simulink library "Vapour_Pressure"  (Simulink 8.2)
settings: Solver=ode45  StartTime=0.0  StopTime=10.0  RelTol=1e-3
undefined symbols (not defined in the file): CarnotCallbacks_Vapour_Pressure
settings Model: Creator=lena.frank  LastModifiedBy=drhf

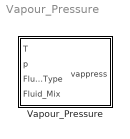
== system Vapour_Pressure ==
  Vapour_Pressure : Subsystem  LoadFcn=CarnotCallbacks_Vapour_Pressure('LoadFcn');  InitFcn=load('THB.mat');  VariantControl=CarlibClassic  mask(vapourpressure){INPUTARGUMENTS=state variables (classic), DEBUGLEVEL=WARNINGLEVEL, MAXTOTALMESSAGES=inf, MAXCONSECUTIVEMESSAGES=inf, WRITETOFILE=0, FILENAME='errors.txt'}
      mask prompts: INPUTARGUMENTS "Input arguments"; DEBUGLEVEL "Debug level"; MAXTOTALMESSAGES "maximum number of total warning"; MAXCONSECUTIVEMESSAGES "maximum number of consecutive warnings"; WRITETOFILE "write messages to file"; FILENAME "filename for error messages"
      mask help:
      | Calculates the vapour pressure of fluids [Pa]. Calls the function "vapourpressure" in the CARNOT library "Carlib".
      | You may use the block "GlobalMessageLevel" in the Toolbox to handle the debugging messages.
      | FluidType        Remarks
      | 1: water          fluid mix is vapourcontent in the 2-phase region
      | 2: air              fluid mix is (kg water) / (kg dry air)
      | 3: cotton oil       function not defined
      | 4: silicone oil     function not defined
      | 5: water-glycol   fluid mix is volume partition [0..1] of propylen glycol
      | 6: Tyfocor LS     function only available in liquid phase
      | 7: Water Constant function not defined
      | 8: Air Constant   function not defined
      mask init:
      | %Inports
      | CarnotCallbacks_Vapour_Pressure('CreateInports');
      | 
      | %global debug level
      | [DEBUGLEVEL, MAXTOTALMESSAGES, MAXCONSECUTIVEMESSAGES, WRITETOFILE, FILENAME] = CarnotCallbacks_Vapour_Pressure('CheckDebugLevels', DEBUGLEVEL, MAXTOTALMESSAGES, MAXCONSECUTIVEMESSAGES, WRITETOFILE, FILENAME);
      mask Help: web(fullfile(path_carnot('help'),'vapourpressure.html'),'-helpbrowser')
      mask TypeOptions INPUTARGUMENTS: state variables (classic) | THB | THV
      mask Callback INPUTARGUMENTS: CarnotCallbacks_Vapour_Pressure('MaskVisibilities');
      mask TypeOptions DEBUGLEVEL: DEBUGLEVEL | INFOLEVEL | WARNINGLEVEL | ERRORLEVEL | FATALLEVEL | NOLEVEL

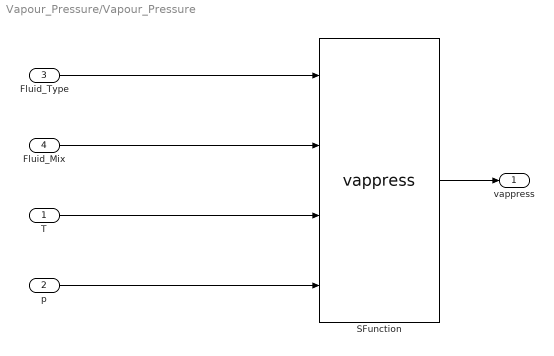
== system Vapour_Pressure/Vapour_Pressure ==
  T : Inport
  p : Inport  Port=2
  Fluid_Type : Inport  Port=3
  Fluid_Mix : Inport  Port=4
  SFunction : S-Function  FunctionName=vappress  Parameters=DEBUGLEVEL,MAXTOTALMESSAGES,MAXCONSECUTIVEMESSAGES,WRITETOFILE,FILENAME  EnableBusSupport=off
  vappress : Outport
  wires:
  SFunction/1 -> vappress/1
  T/1 -> SFunction/3
  p/1 -> SFunction/4
  Fluid_Type/1 -> SFunction/1
  Fluid_Mix/1 -> SFunction/2
